simulink model "proba_real_time_traj"  (R2018b)
settings: Solver=VariableStepAuto  StartTime=0.0  StopTime=100  RelTol=1e-3
values from neighbouring files (symbols this model uses):
  C = -6* acc_min * acc_max ^2 * acc_start^2 * jerk_min ^2 + 6* acc_min^2 * acc_max * acc_end^2 *jerk_min^2 + 12 *  acc_min * jerk_min^2 * jerk_max^2 *vel_max^2    [calculating_trajectory.m]    (also in morus_simulacija_vece_vrijeme_diskretizacije.mat = [1 0 0 0 0 0 0 0 0 1 0 0 ... (64 elements, 8x8)])
  Ts_best = 0.0786839507798    [morus_simulacija_vece_vrijeme_diskretizacije.mat]
undefined symbols (not defined in the file or in its folder): morus_disk
libraries: mpclib x2, robotcorelib x1, robotuavlib x1
settings Model: Creator=branko  LastModifiedBy=branko

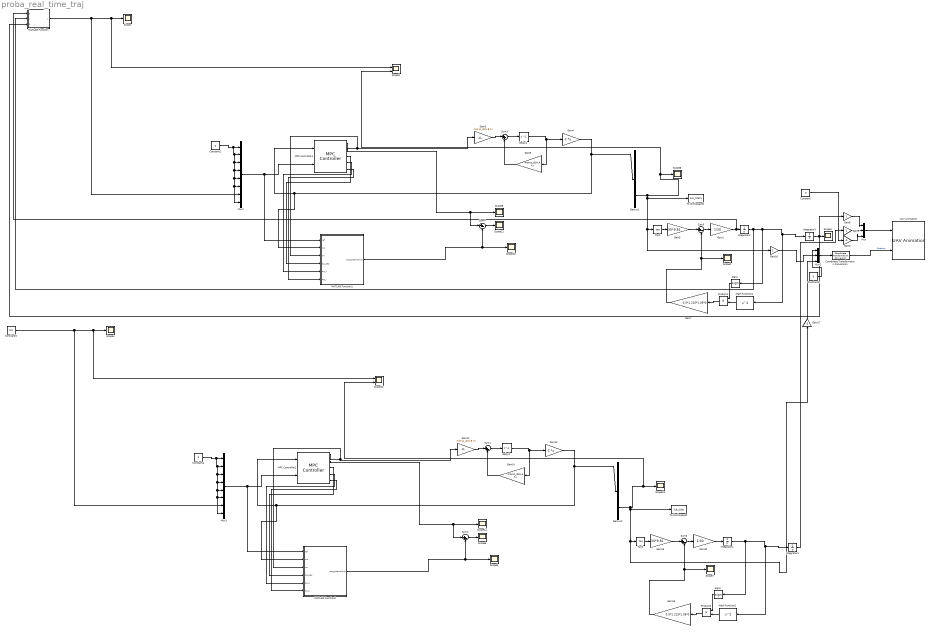
== system proba_real_time_traj ==
  Constant : Constant  Value=0  OutDataTypeStr=double  SampleTime=-1
  Constant1 : Constant  Value=0
  Constant2 : Constant  Value=0  OutDataTypeStr=double  SampleTime=-1
  Constant3 : Constant  Value=0.0  OutDataTypeStr=double  SampleTime=-1
  Constant4 : Constant  Value=0
  Coordinate Transformation Conversion : robotcorelib/Coordinate Transformation Conversion  InputRepresentation=Euler Angles  InputEulerSequence=ZYX  ShowTrVecInputPort=on  OutputRepresentation=Quaternion  OutputEulerSequence=ZYX  ShowTrVecOutputPort=on  SimulateUsing=Code generation
      settings: SourceProductBaseCode=RO
  Delay1 : Delay  DelayLength=1  InitialCondition=0  SampleTime=Ts_best
  Delay2 : Delay  DelayLength=1  InitialCondition=0  SampleTime=Ts_best
  Demux1 : Demux  Outputs=8
  Demux2 : Demux  Outputs=8
  Gain1 : Gain  Gain=1/30
  Gain10 : Gain  Gain=1/30
  Gain11 : Gain  Gain=morus_disk.B  Multiplication=Matrix(K*u)
  Gain12 : Gain  Gain=C  Multiplication=Matrix(K*u)
  Gain13 : Gain  Gain=30*9.81
  Gain14 : Gain  Gain=morus_disk.A  Multiplication=Matrix(K*u)
  Gain15 : Gain  Gain=0.5*1.215*1.05*0
  Gain16 : Gain
  Gain17 : Gain  Gain=-1
  Gain2 : Gain  Gain=-1
  Gain3 : Gain  Gain=morus_disk.B  Multiplication=Matrix(K*u)
  Gain4 : Gain  Gain=C  Multiplication=Matrix(K*u)
  Gain5 : Gain  Gain=30*9.81
  Gain6 : Gain  Gain=morus_disk.A  Multiplication=Matrix(K*u)
  Gain7 : Gain  Gain=0.5*1.215*1.05*0
  Gain8 : Gain
  Gain9 : Gain
  Integrator{1..4} (4 alike) : Integrator
  MATLAB Function : MATLAB Function  TreatAsAtomicUnit=on
  MATLAB Function1 : MATLAB Function  TreatAsAtomicUnit=on
  MATLAB Function2 : MATLAB Function  TreatAsAtomicUnit=on
  MPC Controller1 : mpclib/MPC Controller  SCDEnableBlockLinearizationSpecification=on  mpcobj=mpc1  is_multiple=0  enable_value=0  return_u0=off  updateMPCinCallerWorkspace=on  md_inport=off  mv_inport=off  return_cost=on  return_mvseq=on  return_qpstatus=off  return_xseq=on  return_state=off  return_ovseq=on  state_inport=off  umin_inport=off  umax_inport=off  ymin_inport=off  ymax_inport=off  cc_inport=off  ywt_inport=off  uwt_inport=off  duwt_inport=off  rhoeps_inport=off  uref_inport=off  n_ts=0.078684  n_p=14  n_mv=4  n_md=0  n_ud=0  n_mo=8  n_uo=0  BlockDataType=double  SampleTimeInherited=off  switch_inport=off
  MPC Controller2 : mpclib/MPC Controller  SCDEnableBlockLinearizationSpecification=on  mpcobj=mpc1  is_multiple=0  enable_value=0  return_u0=off  updateMPCinCallerWorkspace=on  md_inport=off  mv_inport=off  return_cost=on  return_mvseq=on  return_qpstatus=off  return_xseq=on  return_state=off  return_ovseq=on  state_inport=off  umin_inport=off  umax_inport=off  ymin_inport=off  ymax_inport=off  cc_inport=off  ywt_inport=off  uwt_inport=off  duwt_inport=off  rhoeps_inport=off  uref_inport=off  n_ts=0.078684  n_p=14  n_mv=4  n_md=0  n_ud=0  n_mo=8  n_uo=0  BlockDataType=double  SampleTimeInherited=off  switch_inport=off
  Math Function1 : Math  Operator=square  SaturateOnIntegerOverflow=on
  Math Function2 : Math  Operator=square  SaturateOnIntegerOverflow=on
  Mux : Mux  Inputs=3
  Mux1 : Mux  Inputs=8
  Mux2 : Mux  Inputs=3
  Mux3 : Mux  Inputs=8
  Product1 : Product
  Product2 : Product
  Scope{,1..2,4..11,13..14} (13 alike) : Scope
  Scope12 : Scope  NumInputPorts=2
  Scope3 : Scope  NumInputPorts=2
  Sign1 : Signum
  Sign2 : Signum
  Sum1 : Sum  Inputs=|++
  Sum{2,4..6} (4 alike) : Sum  Inputs=|+-
  Sum3 : Sum  Inputs=|++
  Tan1 : Trigonometry  Operator=tan
  Tan2 : Trigonometry  Operator=tan
  To Workspace1 : ToWorkspace  VariableName=kut_izlaz1  SaveFormat=Structure With Time  SampleTime=0.01
  To Workspace2 : ToWorkspace  VariableName=kut_izlaz  SaveFormat=Structure With Time  SampleTime=0.01
  UAV Animation : robotuavlib/UAV Animation  UAVType=Multirotor  UAVSize=5  InertialZDirection=Up  SampleTime=1
      settings: SourceProductName=Robotics System Toolbox
  wires:
  MATLAB Function/1(y) -> Mux1/7, Scope3/1, Scope/1
  Gain3/1 -> Sum3/1
  MPC Controller1/4 -> MATLAB Function1/5(op_x)
  MPC Controller1/5 -> MATLAB Function1/6(op_y)
  Delay1/1 -> Gain6/1, Gain4/1
  MPC Controller1/3 -> MATLAB Function1/4(op_seq)
  Gain6/1 -> Sum3/2
  Gain7/1 -> Scope2/1, Sum5/2
  Integrator2/1 -> MATLAB Function/2(v), Sign1/1, Math Function1/1, Integrator3/1
  Math Function1/1 -> Product1/2
  MPC Controller1/1 -> MATLAB Function1/3(mv), Gain3/1
  MATLAB Function1/1(cost_alternative) -> Scope10/1, Sum4/2
  Sum3/1 -> Delay1/1
  Gain4/1 -> MATLAB Function1/2(mo), MPC Controller1/1, Demux1/1
  Sum4/1 -> Scope11/1
  Gain5/1 -> Sum5/1
  Sign1/1 -> Product1/1
  Tan1/1 -> Gain5/1
  Constant1/1 -> Mux1/8, Mux1/6, Mux1/5, Mux1/4, Mux1/3, Mux1/2, Mux1/1
  MPC Controller1/2 -> Sum4/1, Scope9/1
  Product1/1 -> Gain7/1
  Mux1/1 -> MATLAB Function1/1(ref), MPC Controller1/2
  Sum5/1 -> Gain1/1
  Gain1/1 -> MATLAB Function/1(a), Integrator2/1
  Gain2/1 -> Mux/3
  Mux/1 -> UAV Animation/1
  Gain8/1 -> Mux/1
  Integrator3/1 -> Gain8/1, MATLAB Function/3(p), Scope1/1
  Coordinate Transformation Conversion/1 -> UAV Animation/2  "Rotation"
  Gain9/1 -> Mux/2
  Mux2/1 -> Coordinate Transformation Conversion/1
  Constant/1 -> Gain2/1
  Constant2/1 -> Mux2/1
  Demux1/7 -> To Workspace1/1, Gain16/1, Tan1/1, Scope3/2, Scope8/1
  Sum6/1 -> Gain10/1
  Tan2/1 -> Gain13/1
  Gain10/1 -> Integrator1/1
  Sign2/1 -> Product2/1
  Mux3/1 -> MATLAB Function2/1(ref), MPC Controller2/2
  Sum1/1 -> Delay2/1
  Product2/1 -> Gain15/1
  MPC Controller2/2 -> Sum2/1, Scope14/1
  Constant4/1 -> Mux3/8, Mux3/6, Mux3/5, Mux3/4, Mux3/3, Mux3/2, Mux3/1
  Delay2/1 -> Gain14/1, Gain12/1
  Gain13/1 -> Sum6/1
  Constant3/1 -> Mux3/7, Scope12/1, Scope4/1
  MPC Controller2/3 -> MATLAB Function2/4(op_seq)
  Math Function2/1 -> Product2/2
  MPC Controller2/5 -> MATLAB Function2/6(op_y)
  Demux2/7 -> To Workspace2/1, Gain17/1, Tan2/1, Scope12/2, Scope13/1
  Gain12/1 -> MATLAB Function2/2(mo), MPC Controller2/1, Demux2/1
  Gain15/1 -> Scope7/1, Sum6/2
  MPC Controller2/1 -> MATLAB Function2/3(mv), Gain11/1
  MPC Controller2/4 -> MATLAB Function2/5(op_x)
  Gain14/1 -> Sum1/2
  MATLAB Function2/1(cost_alternative) -> Scope5/1, Sum2/2
  Integrator1/1 -> Sign2/1, Math Function2/1, Integrator4/1
  Gain11/1 -> Sum1/1
  Sum2/1 -> Scope6/1
  Integrator4/1 -> Gain9/1
  Gain16/1 -> Mux2/2
  Gain17/1 -> Mux2/3

== matlab function proba_real_time_traj/MATLAB Function1 ==
  data: ref input; cost_alternative output; mo input; mv input; op_seq input; op_x input; op_y input
function cost_alternative = fcn(ref, mo, mv, op_seq, op_x, op_y)
all_ref = repmat(ref,1,size(op_y,1)-1);

S_mv = diag([0.58,0.58, 100, 100]);
S_ov = diag([0.58, 4, 0.58, 4, 800, 800, 0.5236,0.5236]);

e_y = (S_ov)\( (op_y(2:end,:)' - all_ref));
e_u = (S_mv)\((- op_seq(2:end,:)'));
e_du = (S_mv)\((op_seq(2:end,:)' - op_seq(1:end-1,:)'));


MV_weights = diag( [0.406005849709838 0.406005849709838 0 0]).^2;
MVRate_weight=  diag([0.0738905609893065 0.0738905609893065 0.0738905609893065 0.0738905609893065]).^2;
OutputVariables=diag([1.0826822658929 0 1.0826822658929 0 0 0 0.270670566473225 0.135335283236613]).^2;
ECR = 100000;
lol1 = e_y .*(OutputVariables *e_y);
lol2 = e_u .* (MV_weights *e_u);
lol3 = e_du .* (MVRate_weight *e_du);
cost_alternative =sum(sum(lol3,'double'), 'double')+sum(sum(lol2,'double'), 'double')+sum(sum(lol1,'double'), 'double') ;
end

== matlab function proba_real_time_traj/MATLAB Function2 ==
  data: ref input; cost_alternative output; mo input; mv input; op_seq input; op_x input; op_y input
function cost_alternative = fcn(ref, mo, mv, op_seq, op_x, op_y)
all_ref = repmat(ref,1,size(op_y,1)-1);

S_mv = diag([0.58,0.58, 100, 100]);
S_ov = diag([0.58, 4, 0.58, 4, 800, 800, 0.5236,0.5236]);

e_y = (S_ov)\( (op_y(2:end,:)' - all_ref));
e_u = (S_mv)\((- op_seq(2:end,:)'));
e_du = (S_mv)\((op_seq(2:end,:)' - op_seq(1:end-1,:)'));


MV_weights = diag( [0.406005849709838 0.406005849709838 0 0]).^2;
MVRate_weight=  diag([0.0738905609893065 0.0738905609893065 0.0738905609893065 0.0738905609893065]).^2;
OutputVariables=diag([1.0826822658929 0 1.0826822658929 0 0 0 0.270670566473225 0.135335283236613]).^2;
ECR = 100000;
lol1 = e_y .*(OutputVariables *e_y);
lol2 = e_u .* (MV_weights *e_u);
lol3 = e_du .* (MVRate_weight *e_du);
cost_alternative =sum(sum(lol3,'double'), 'double')+sum(sum(lol2,'double'), 'double')+sum(sum(lol1,'double'), 'double') ;
end

== matlab function proba_real_time_traj/MATLAB Function ==
  settings: updateMethod=DISCRETE  sampleTime=0.1
  data: a input size=1; y output size=1; v input size=1; p input size=1
function y = fcn(a,v,p)
jerk_max = 1;
jerk_min = -1;
acc_max = 0.5; 
acc_min = -0.5;
vel_max  = 1;
vel_min = -1;
vel_start = v; 
vel_end = 0;
p_start  =p;
p_end = 20;
acc_start =a ;
acc_end = 0;
theta = 0.0;
timer = 0.0;
[theta, timer] = calculate_theta_simulink(jerk_max, jerk_min, acc_max, acc_min,vel_max,vel_min, vel_start, vel_end ,p_start , p_end , acc_start, acc_end );
if(isempty(theta))
    theta = 0.0;
end
y = theta(1);
end
